simulink model "Controller"  (Simulink 10.0)
settings: Solver=FixedStepAuto  StartTime=0.0  StopTime=10.0  RelTol=1e-3
values from neighbouring files (symbols this model uses):
  Controlador = Simulink.Parameter    [Param_Controller.m]
  userParameters = Simulink.Parameter    [Param_Controller.m]
undefined symbols (not defined in the file or in its folder): Controlador_Curva, controllerGainsCurve, ControllerState_t, filter_r_den, filter_r_num, filter_r_Ts
libraries: simulink x8
settings Model: Creator=renan  LastModifiedBy=renan
settings DataIOCC: SaveFormat=Dataset  ReturnWorkspaceOutputs=on
settings OptimizationCC: DefaultParameterBehavior=Inlined  UseFloatMulNetSlope=on  DefaultUnderspecifiedDataType=single  PassReuseOutputArgsAs=Individual arguments  LifeSpan=auto  OptimizationLevel=level1  OptimizationPriority=Speed  MultiThreadedLoops=on  EfficientTunableParamExpr=on
settings DebuggingCC: UnderspecifiedInitializationDetection=Simplified  MergeDetectMultiDrivingBlocksExec=error  ParameterTunabilityLossMsg=error  SFUnexpectedBacktrackingDiag=error  SFNoUnconditionalDefaultTransitionDiag=error  SFExecutionAtInitializationDiag=warning  ArithmeticOperatorsInVariantConditions=error
settings HardwareCC: ProdBitPerPointer=64  ProdBitPerSizeT=64  ProdBitPerPtrDiffT=64  ProdLargestAtomicFloat=Float  ProdIntDivRoundTo=Zero  ProdEndianess=LittleEndian  ProdWordSize=64  ProdLongLongMode=on  ProdHWDeviceType=Intel->x86-64 (Windows64)
settings ModelReferenceCC: PropagateSignalLabelsOutOfModel=on
settings SFSimCC: SimUseLocalCustomCode=on  MATLABDynamicMemAlloc=off  CustomCodeUndefinedFunction=FilterOut
settings RTWCC: Description=Embedded Coder  SystemTargetFile=ert.tlc  TemplateMakefile=ert_default_tmf  GenerateReport=on  RTWUseLocalCustomCode=on  Toolchain=MinGW64 | gmake (64-bit Windows)  IncludeHyperlinkInReport=on  LaunchReport=on  TargetLang=C++  GenerateTraceInfo=on  GenerateTraceReport=on  GenerateTraceReportSl=on  GenerateTraceReportSf=on  GenerateTraceReportEml=on
settings CodeAppCC: ForceParamTrailComments=on  IgnoreCustomStorageClasses=off  OperatorAnnotations=on  SimulinkDataObjDesc=on  SFDataObjDesc=on  InsertBlockDesc=on  StateflowObjectComments=off
settings ERTTargetCC: TargetLangStandard=C++03 (ISO)  GenerateSampleERTMain=on  SuppressErrorStatus=on  MultiInstanceERTCode=on  CodeInterfacePackaging=C++ class  SupportNonFinite=off  SupportComplex=off  RootIOFormat=Structure reference  ERTCustomFileTemplate=example_file_process.tlc
settings CPPComponent: GenerateDestructor=on  GenerateExternalIOAccessMethods=None  ParameterMemberVisibility=public  InternalMemberVisibility=private  GenerateParameterAccessMethods=None  GenerateInternalMemberAccessMethods=None  UseOperatorNewForModelRefRegistration=off
settings ConfigComp: CovMetricSettings=dwe  CovHtmlReporting=off  CovSaveCumulativeToWorkspaceVar=off  CovSaveSingleToWorkspaceVar=off

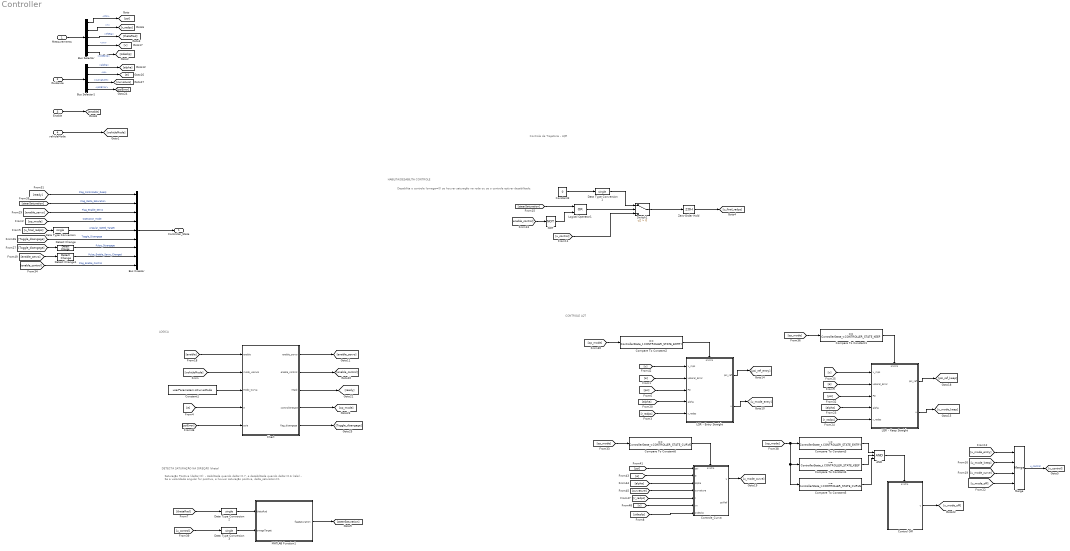
== system Controller ==
  note: DETECTA SATURAÇÃO NA DIREÇÃO (theta)
  note: LOGICA
  note: Desabilita o controle (omega=0) se houver saturação na roda ou se o controle estiver desabilitado.
  note: Controle de Trajetória - LQR
  note: Saturação Positiva (delta>0):
      | - Habilitada quando delta>0.7, e desabilitada quando delta<0.6 (relé)
      | - Se a velocidade angular for positiva, e houver saturação positiva, delta_saturation=1
  note: CONTROLE LQT
  note: HABILITA/DESABILITA CONTROLE
  Measurements : Inport  OutDataTypeStr=Bus: controllerMeasurementBus_t
  Guidance : Inport  Port=2  OutDataTypeStr=Bus: controllerInputGuidanceBus_t
  Enable : Inport  Port=3  OutDataTypeStr=boolean
  vehicleMode : Inport  Port=4  OutDataTypeStr=Enum: VehicleMode_t
  AND : Logic  Inputs=3  IconShape=distinctive  AllPortsSameDT=off  OutDataTypeStr=boolean
  Bus Creator : BusCreator  Inputs=9  OutDataTypeStr=Bus: Controler_Bus  NonVirtualBus=on
  Bus Selector : BusSelector  OutputSignals=Psi,r,theta,vx,sideslip
  Bus Selector1 : BusSelector  OutputSignals=alpha,e,curvature,psiError
  Chart : Stateflow chart  BlockKeywords=__PRM__SERIALIZED__DATA__:Stateflow Chart,Stateflow Diagram  TreatAsAtomicUnit=on
  Compare To Constant1 : simulink/Logic and Bit Operations/Compare To Constant  relop===  const=ControllerState_t.CONTROLLER_STATE_KEEP  OutDataTypeStr=boolean
  Compare To Constant2 : simulink/Logic and Bit Operations/Compare To Constant  relop===  const=ControllerState_t.CONTROLLER_STATE_ENTRY  OutDataTypeStr=boolean
  Compare To Constant3 : simulink/Logic and Bit Operations/Compare To Constant  relop=~=  const=ControllerState_t.CONTROLLER_STATE_ENTRY  OutDataTypeStr=boolean
  Compare To Constant4 : simulink/Logic and Bit Operations/Compare To Constant  relop=~=  const=ControllerState_t.CONTROLLER_STATE_KEEP  OutDataTypeStr=boolean
  Compare To Constant5 : simulink/Logic and Bit Operations/Compare To Constant  relop=~=  const=ControllerState_t.CONTROLLER_STATE_CURVE  OutDataTypeStr=boolean
  Compare To Constant6 : simulink/Logic and Bit Operations/Compare To Constant  relop===  const=ControllerState_t.CONTROLLER_STATE_CURVE  OutDataTypeStr=boolean
  Constant1 : Constant  Value=userParameters.isCurveMode
  Constant3 : Constant  Value=0
  Control Off : Subsystem  TreatAsAtomicUnit=on
  Controle_Curva : Subsystem  TreatAsAtomicUnit=on
  Data Type Conversion{,1..3} (4 alike) : DataTypeConversion  OutDataTypeStr=single
  Detect Change : simulink/Logic and Bit Operations/Detect Change  vinit=0  OutDataTypeStr=boolean
  Detect Change1 : simulink/Logic and Bit Operations/Detect Change  vinit=0  OutDataTypeStr=boolean
  LQR - Entry Straight : Subsystem  TreatAsAtomicUnit=on
  LQR - Keep Straight : Subsystem  TreatAsAtomicUnit=on
  Logical Operator1 : Logic  Operator=OR  IconShape=distinctive  AllPortsSameDT=off  OutDataTypeStr=boolean
  MATLAB Function1 : MATLAB Function  TreatAsAtomicUnit=on
  Merge : Merge  Inputs=4  InitialOutput=0
  NOT : Logic  Operator=NOT  IconShape=distinctive  AllPortsSameDT=off  OutDataTypeStr=boolean
  Switch1 : Switch  Criteria=u2 > Threshold
  Zero-Order Hold : ZeroOrderHold  SampleTime=0.05
  Controller_State : Outport  OutDataTypeStr=Bus: Controler_Bus
  wires:
  [r_radps] -> LQR - Entry Straight/5(r_radps)
  Compare To Constant5/1 -> AND/3
  [psiError] -> Chart/5(psie)
  [u_mode_keep] -> Merge/2
  LQR - Keep Straight/2(u) -> [u_mode_keep]
  Compare To Constant4/1 -> AND/2
  [Toggle_disengage] -> Detect Change/1
  [v] -> Controle_Curva/6(vx)
  Detect Change1/1 -> Bus Creator/8  "Pulse_Enable_Servo_Changed"
  Detect Change/1 -> Bus Creator/7  "Pulse_Disengage"
  LQR - Entry Straight/2(u) -> [u_mode_entry]
  [Toggle_disengage] -> Bus Creator/6  "Toggle_Disengage"
  [enable_servo] -> Detect Change1/1
  [enable_servo] -> Bus Creator/3  "Flag_Enable_Servo"
  Merge/1 -> [u_control]  "u_control"
  Chart/3(ready) -> [ready]
  [r_radps] -> Controle_Curva/5(r)
  [op_mode] -> Bus Creator/4  "Operation_Mode"
  [u_final_radps] -> Data Type Conversion/1
  [alpha] -> Controle_Curva/3(alpha)
  [psi] -> Controle_Curva/1(psi)
  Data Type Conversion/1 -> Bus Creator/5  "Angular_Speed_Target"
  [e] -> Controle_Curva/2(e)
  [op_mode] -> Compare To Constant6/1
  [steerSaturation] -> Bus Creator/2  "Flag_Delta_Saturation"
  Compare To Constant3/1 -> AND/1
  Bus Creator/1 -> Controller_State/1
  Compare To Constant2/1 -> LQR - Entry Straight/Enable
  Constant1/1 -> Chart/3(Modo_Curva)
  [u_control] -> Switch1/3
  [u_mode_entry] -> Merge/1
  [u_mode_off] -> Merge/4
  [e] -> Chart/4(e)
  [e] -> LQR - Entry Straight/2(Lateral_Error)
  Control Off/1(u) -> [u_mode_off]
  [ready] -> Bus Creator/1  "Flag_Controlador_Ready"
  Chart/5(flag_disengage) -> [Toggle_disengage]
  [psi] -> LQR - Entry Straight/3(Psi)
  [u_mode_curve] -> Merge/3
  Compare To Constant6/1 -> Controle_Curva/Enable
  LQR - Entry Straight/1(psi_ref) -> [psi_ref_entry]
  Switch1/1 -> Zero-Order Hold/1
  [v] -> LQR - Entry Straight/1(v_mps)
  Compare To Constant1/1 -> LQR - Keep Straight/Enable
  [psi] -> LQR - Keep Straight/3(Psi)
  AND/1 -> Control Off/Enable
  [op_mode] -> Compare To Constant5/1, Compare To Constant4/1, Compare To Constant3/1
  [r_radps] -> LQR - Keep Straight/5(r_radps)
  [v] -> LQR - Keep Straight/1(v_mps)
  [e] -> LQR - Keep Straight/2(Lateral_Error)
  [alpha] -> LQR - Entry Straight/4(alpha)
  [op_mode] -> Compare To Constant1/1
  [steerSaturation] -> Logical Operator1/1
  [op_mode] -> Compare To Constant2/1
  Controle_Curva/1(u) -> [u_mode_curve]
  Logical Operator1/1 -> Switch1/2
  Chart/1(enable_servo) -> [enable_servo]
  [curvature] -> Controle_Curva/4(curvature)
  [alpha] -> LQR - Keep Straight/4(alpha)
  Chart/4(controllerState) -> [op_mode]
  Chart/2(enable_control) -> [enable_control]
  NOT/1 -> Logical Operator1/2
  Constant3/1 -> Data Type Conversion1/1
  [enable] -> Chart/1(enable)
  LQR - Keep Straight/1(psi_ref) -> [psi_ref_keep]
  [enable_control] -> NOT/1
  Bus Selector/1 -> [psi]  "<Psi>"
  Bus Selector/2 -> [r_radps]  "<r>"
  Bus Selector/3 -> [thetaRad]  "<theta>"
  Bus Selector/4 -> [v]  "<vx>"
  Guidance/1 -> Bus Selector1/1
  Bus Selector1/1 -> [alpha]  "<alpha>"
  Bus Selector1/2 -> [e]  "<e>"
  Bus Selector1/3 -> [curvature]  "<curvature>"
  [enable_control] -> Bus Creator/9  "Flag_Enable_Control"
  Data Type Conversion1/1 -> Switch1/1
  Zero-Order Hold/1 -> [u_final_radps]
  MATLAB Function1/1(flagSaturation) -> [steerSaturation]
  [thetaRad] -> Data Type Conversion2/1
  [u_control] -> Data Type Conversion3/1
  Data Type Conversion2/1 -> MATLAB Function1/1(thetaRad)
  Data Type Conversion3/1 -> MATLAB Function1/2(omegaTarget)
  Bus Selector1/4 -> [psiError]  "<psiError>"
  Enable/1 -> [enable]
  vehicleMode/1 -> [vehicleMode]
  [vehicleMode] -> Chart/2(modo_veiculo)
  Measurements/1 -> Bus Selector/1
  Bus Selector/5 -> [sideslip]  "<sideslip>"
  [sideslip] -> Controle_Curva/7(sideslip)

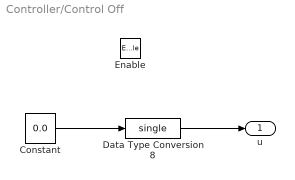
== system Controller/Control Off ==
  Enable : EnablePort
  Constant : Constant  Value=0.0  OutDataTypeStr=single  SampleTime=-1
  Data Type Conversion8 : DataTypeConversion  OutDataTypeStr=single
  u : Outport
  wires:
  Constant/1 -> Data Type Conversion8/1
  Data Type Conversion8/1 -> u/1

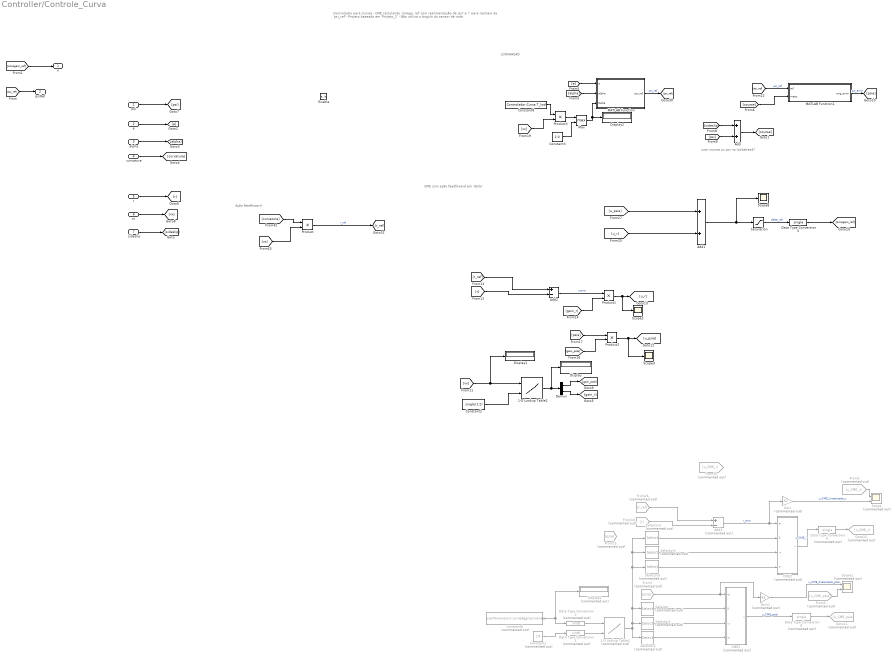
== system Controller/Controle_Curva ==
  note: usar course ou psi no lookahead?
  note: Controlador para Curvas
      |
      | - CME calculando 'omega_ref' com realimentação de 'psi' e 'r' para rastreio de 'psi_ref'
      | - Projeto baseado em 'Projeto_2'
      | - Não utiliza o ângulo do sensor de roda
  note: LOOKAHEAD
  note: CME com ação feedfoward em 'delta'
  note: Ação feedfoward
  psi : Inport  OutDataTypeStr=single  PortDimensions=1
  e : Inport  Port=2  OutDataTypeStr=single  PortDimensions=1
  alpha : Inport  Port=3  OutDataTypeStr=single  PortDimensions=1
  curvature : Inport  Port=4  OutDataTypeStr=single  PortDimensions=1
  r : Inport  Port=5  OutDataTypeStr=single  PortDimensions=1
  vx : Inport  Port=6  OutDataTypeStr=single  PortDimensions=1
  sideslip : Inport  Port=7
  Enable : EnablePort
  1-D Lookup Table1 : Lookup_n-D  Commented=on  BreakpointsForDimension1=uint8(1:7)  BreakpointsForDimension2=uint8(1:8)  IndexSearchMethod=Linear search  BeginIndexSearchUsingPreviousIndexResult=on  Table=controllerGainsCurve  ExtrapMethod=Clip  UseLastTableValue=on  InternalRulePriority=Speed  OutDataTypeStr=single  RndMeth=Simplest  InputSameDT=on
  1-D Lookup Table2 : Lookup_n-D  BreakpointsForDimension1=Controlador.Curva.v_index  BreakpointsForDimension2=uint8(1:2)  IndexSearchMethod=Linear search  BeginIndexSearchUsingPreviousIndexResult=on  Table=Controlador.Curva.Gains  ExtrapMethod=Clip  UseLastTableValue=on  InternalRulePriority=Speed  OutDataTypeStr=single  RndMeth=Simplest  InputSameDT=on
  Add : Sum
  Add1 : Sum
  Add2 : Sum  Inputs=+-
  Add3 : Sum  Commented=on  Inputs=+-
  CME1 : MATLAB Function  Commented=on  TreatAsAtomicUnit=on
  CME2 : MATLAB Function  Commented=on  TreatAsAtomicUnit=on
  Constant1 : Constant  Commented=on  Value=1:8
  Constant2 : Constant  Value=single(1:2)
  Constant3 : Constant  Value=2.0
  Constant6 : Constant  Commented=on  Value=userParameters.curveAggressiveness
  Constant8 : Constant  Value=Controlador.Curva.T_look  SampleTime=-1
  Data Type Conversion1 : DataTypeConversion  Commented=on  OutDataTypeStr=uint8
  Data Type Conversion2 : DataTypeConversion  Commented=on  OutDataTypeStr=uint8
  Data Type Conversion3 : DataTypeConversion  OutDataTypeStr=single
  Data Type Conversion8 : DataTypeConversion  Commented=on  OutDataTypeStr=single
  Data Type Conversion9 : DataTypeConversion  Commented=on  OutDataTypeStr=single
  Demux : Demux  Outputs=2
  Display : Display
  Display1 : Display
  Display2 : Display
  Display4 : Display  Commented=on
  From15 : From  Commented=on  GotoTag=psie
  From16 : From  Commented=on  GotoTag=r
  From2 : From  Commented=on  GotoTag=u_CME_r
  From20 : From  Commented=on  GotoTag=u_CME_r
  From26 : From  Commented=on  GotoTag=r_ref
  From3 : From  Commented=on  GotoTag=u_CME_psie
  From7 : From  Commented=on  GotoTag=psie
  Gain : Gain  Commented=on  Gain=52
  Gain1 : Gain  Commented=on  Gain=43
  Goto11 : Goto  Commented=on  GotoTag=u_CME_psie
  Goto15 : Goto  Commented=on  GotoTag=u_CME_r
  MATLAB Function : MATLAB Function  TreatAsAtomicUnit=on
  MATLAB Function1 : MATLAB Function  TreatAsAtomicUnit=on
  Max : MinMax  Function=max  Inputs=2
  Product{,1..3} (4 alike) : Product
  Saturation : Saturate  UpperLimit=Controlador.Curva.omegam_sat  LowerLimit=-Controlador.Curva.omegam_sat
  Scope : Scope  Commented=on  NumInputPorts=2
  Scope1 : Scope  Commented=on  NumInputPorts=2
  Scope2 : Scope
  Scope3 : Scope
  Scope8 : Scope
  Selector : Selector  Commented=on  InputPortWidth=8  IndexOptions=Index vector (dialog)  Indices=[2]  OutputSizes=1
  Selector1 : Selector  Commented=on  InputPortWidth=8  IndexOptions=Index vector (dialog)  Indices=[3 4]  OutputSizes=1
  Selector2 : Selector  Commented=on  InputPortWidth=8  IndexOptions=Index vector (dialog)  Indices=[1]  OutputSizes=1
  Selector3 : Selector  Commented=on  InputPortWidth=8  IndexOptions=Index vector (dialog)  Indices=[6]  OutputSizes=1
  Selector4 : Selector  Commented=on  InputPortWidth=8  IndexOptions=Index vector (dialog)  Indices=[7 8]  OutputSizes=1
  Selector5 : Selector  Commented=on  InputPortWidth=8  IndexOptions=Index vector (dialog)  Indices=[5]  OutputSizes=1
  u : Outport
  psiRef : Outport  Port=2
  wires:
  [psi_ref] -> MATLAB Function1/1(ref)  "psi_ref"
  MATLAB Function/1(psi_ref) -> [psi_ref]  "psi_ref"
  MATLAB Function1/1(ang_error) -> [psie]  "psi_error"
  [e] -> MATLAB Function/1(e)
  [alpha] -> MATLAB Function/2(alpha)
  Add1/1 -> Scope8/1, Saturation/1
  CME2/1(u) -> Data Type Conversion9/1  "u_CME_r"
  CME1/1(u) -> Data Type Conversion8/1  "u_CME_psie"
  From26/1 -> Add3/1
  From16/1 -> Add3/2
  Saturation/1 -> Data Type Conversion3/1  "delta_ref"
  Product/1 -> [r_ref]  "r_ref"
  [curvature] -> Product/1
  [vx] -> Product/2
  psi/1 -> [psi]
  e/1 -> [e]
  alpha/1 -> [alpha]
  curvature/1 -> [curvature]
  r/1 -> [r]
  Add3/1 -> Gain/1, CME2/1(et)  "r_erro"
  [omegam_ref] -> u/1
  vx/1 -> [vx]
  From7/1 -> CME1/1(et), Gain1/1
  Selector/1 -> CME1/2(B)
  Selector1/1 -> CME1/3(ur)
  Selector2/1 -> CME1/4(er)
  Selector3/1 -> CME2/2(B)
  Selector4/1 -> CME2/3(ur)
  Selector5/1 -> CME2/4(er)
  Data Type Conversion8/1 -> Goto11/1
  Data Type Conversion9/1 -> Goto15/1
  Gain/1 -> Scope/2  "u_CME_Linearizado_r"
  Gain1/1 -> Scope1/1  "u_CME_linearizado_psie"
  Constant6/1 -> Display4/1, Data Type Conversion2/1
  Constant1/1 -> Data Type Conversion1/1
  1-D Lookup Table1/1 -> Selector3/1, Selector4/1, Selector5/1, Selector/1, Selector1/1, Selector2/1
  Data Type Conversion2/1 -> 1-D Lookup Table1/1
  Data Type Conversion1/1 -> 1-D Lookup Table1/2
  [psi_ref] -> psiRef/1
  From2/1 -> Scope/1
  From3/1 -> Scope1/2
  sideslip/1 -> [sideslip]
  [sideslip] -> Add/1
  [psi] -> Add/2
  Add/1 -> [course]
  [vx] -> Display1/1, 1-D Lookup Table2/1
  Constant2/1 -> 1-D Lookup Table2/2
  1-D Lookup Table2/1 -> Display/1, Demux/1
  Demux/1 -> [gain_psie]
  Demux/2 -> [gain_r]
  [r_ref] -> Add2/1
  Add2/1 -> Product1/1  "r_erro"
  [r] -> Add2/2
  [psie] -> Product2/1
  Product2/1 -> Scope3/1, [u_psie]
  Product1/1 -> Scope2/1, [u_r]
  Constant8/1 -> Product3/1
  [vx] -> Product3/2
  Product3/1 -> Max/1
  Max/1 -> Display2/1, MATLAB Function/3(Delta)
  Constant3/1 -> Max/2
  [u_psie] -> Add1/1
  [u_r] -> Add1/2
  [gain_psie] -> Product2/2
  [gain_r] -> Product1/2
  [course] -> MATLAB Function1/2(meas)
  Data Type Conversion3/1 -> [omegam_ref]

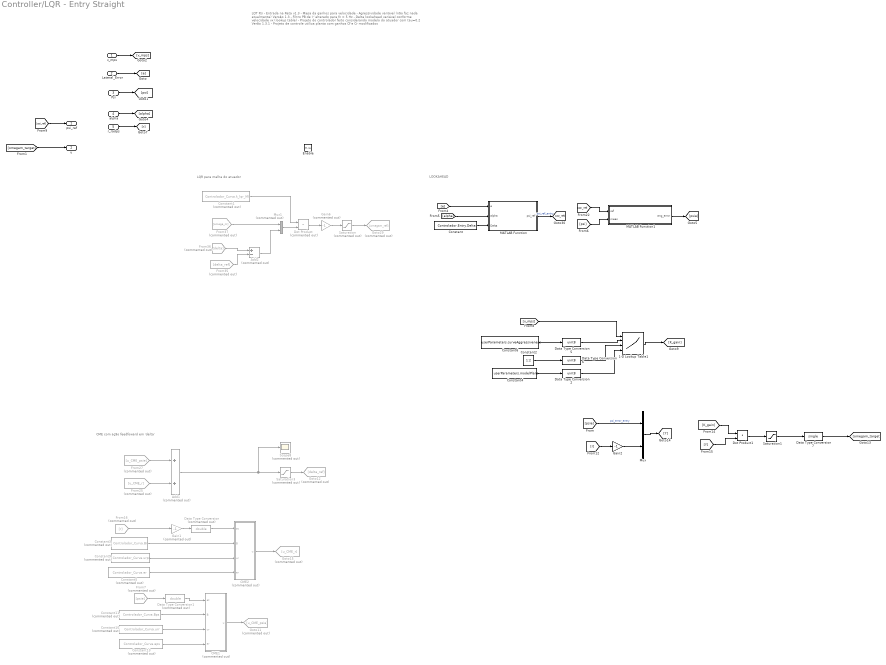
== system Controller/LQR - Entry Straight ==
  note: LQT Psi - Entrada na Reta v1.3
      | - Mapa da ganhos para velocidade
      | - Agressividade variável (não faz nada atualmente)
      |
      | Versão 1.3
      | - Filtro PB de 'r' alterado para fc = 5 Hz
      | - Delta lookahead variável conforme velocidade vx (lookup table)
      | - Projeto do controlador feito considerando modelo do atuador com tau=0.2
      |
      | Verão 1.3.1
      | - Projeto de controle utiliza planta com ganhos Cf e Cr modificados
  note: LQR para malha do atuador
  note: LOOKAHEAD
  note: CME com ação feedfoward em 'delta'
  v_mps : Inport  OutDataTypeStr=single  PortDimensions=1
  Lateral_Error : Inport  Port=2  PortDimensions=1
  Psi : Inport  Port=3  PortDimensions=1
  alpha : Inport  Port=4  PortDimensions=1
  r_radps : Inport  Port=5  PortDimensions=1
  Enable : EnablePort
  1-D Lookup Table1 : Lookup_n-D  NumberOfTableDimensions=4  BreakpointsForDimension1=Controlador.Entry.v_index  BreakpointsForDimension2=uint8(1:7)  BreakpointsForDimension3=uint8(1:2)  BreakpointsForDimension4=uint8(1:2)  IndexSearchMethod=Linear search  BeginIndexSearchUsingPreviousIndexResult=on  Table=Controlador.Entry.Gains  TableDataTypeStr=Inherit: Inherit from 'Table data'  ExtrapMethod=Clip  UseLastTableValue=on  InternalRulePriority=Speed  OutDataTypeStr=Inherit: Inherit from 'Table data'  RndMeth=Simplest
  Add1 : Sum  Commented=on
  Add2 : Sum  Commented=on  Inputs=+-
  CME1 : MATLAB Function  Commented=on  TreatAsAtomicUnit=on
  CME2 : MATLAB Function  Commented=on  TreatAsAtomicUnit=on
  Constant : Constant  Value=Controlador.Entry.Delta
  Constant1 : Constant  Commented=on  Value=Controlador_Curva.k_lqr_MI  VectorParams1D=off  SampleTime=-1
  Constant10 : Constant  Commented=on  Value=Controlador_Curva.urr  VectorParams1D=off  SampleTime=-1
  Constant11 : Constant  Commented=on  Value=Controlador_Curva.Bps  SampleTime=-1
  Constant13 : Constant  Commented=on  Value=Controlador_Curva.eps  SampleTime=-1
  Constant2 : Constant  Value=1:2
  Constant3 : Constant  Commented=on  Value=Controlador_Curva.Br  SampleTime=-1
  Constant4 : Constant  Value=userParameters.modelPlant
  Constant5 : Constant  Commented=on  Value=Controlador_Curva.er  SampleTime=-1
  Constant6 : Constant  Value=userParameters.curveAggressiveness
  Constant9 : Constant  Commented=on  Value=Controlador_Curva.urps  VectorParams1D=off  SampleTime=-1
  Data Type Conversion : DataTypeConversion  Commented=on  OutDataTypeStr=double
  Data Type Conversion1 : DataTypeConversion  Commented=on  OutDataTypeStr=double
  Data Type Conversion2 : DataTypeConversion  OutDataTypeStr=uint8
  Data Type Conversion5 : DataTypeConversion  OutDataTypeStr=uint8
  Data Type Conversion6 : DataTypeConversion  OutDataTypeStr=uint8
  Data Type Conversion7 : DataTypeConversion  OutDataTypeStr=single
  Dot Product : DotProduct  Commented=on  InputSameDT=on  OutDataTypeStr=Inherit: Inherit via internal rule
  Dot Product1 : DotProduct  InputSameDT=on  OutDataTypeStr=Inherit: Inherit via internal rule
  From16 : From  Commented=on  GotoTag=r
  From25 : From  Commented=on  GotoTag=u_CME_r
  From27 : From  Commented=on  GotoTag=u_CME_psie
  From35 : From  Commented=on  GotoTag=delta_ref
  From36 : From  Commented=on  GotoTag=delta
  From37 : From  Commented=on  GotoTag=omega_m
  From7 : From  Commented=on  GotoTag=psie
  Gain1 : Gain  Commented=on  Gain=-1
  Gain2 : Gain  Gain=-1
  Gain6 : Gain  Commented=on  Gain=-1
  Goto11 : Goto  Commented=on  GotoTag=u_CME_psie
  Goto12 : Goto  Commented=on  GotoTag=delta_ref
  Goto15 : Goto  Commented=on  GotoTag=u_CME_r
  Goto29 : Goto  Commented=on  GotoTag=omegam_ref
  MATLAB Function : MATLAB Function  TreatAsAtomicUnit=on
  MATLAB Function1 : MATLAB Function  TreatAsAtomicUnit=on
  Mux : Mux  Inputs=2
  Mux1 : Mux  Commented=on  Inputs=2
  Saturation : Saturate  Commented=on  UpperLimit=4  LowerLimit=-4
  Saturation1 : Saturate  UpperLimit=Controlador.Entry.omegam_sat  LowerLimit=-Controlador.Entry.omegam_sat
  Saturation3 : Saturate  Commented=on  UpperLimit=0.8  LowerLimit=-0.8
  Scope8 : Scope  Commented=on
  psi_ref : Outport
  u : Outport  Port=2
  wires:
  v_mps/1 -> [v_mps]
  Lateral_Error/1 -> [e]
  Psi/1 -> [psi]
  alpha/1 -> [alpha]
  r_radps/1 -> [r]
  [psi_ref] -> psi_ref/1
  [e] -> MATLAB Function/1(e)
  From35/1 -> Add2/2
  Add2/1 -> Mux1/2
  Constant10/1 -> CME1/3(ur)
  Data Type Conversion/1 -> CME2/1(et)
  Saturation3/1 -> Goto12/1
  Mux1/1 -> Dot Product/2
  Constant3/1 -> CME2/2(B)
  Gain6/1 -> Saturation/1
  Dot Product/1 -> Gain6/1
  From37/1 -> Mux1/1
  From36/1 -> Add2/1
  Constant9/1 -> CME2/3(ur)
  Saturation/1 -> Goto29/1
  From27/1 -> Add1/1
  Constant11/1 -> CME1/2(B)
  Constant1/1 -> Dot Product/1
  From16/1 -> Gain1/1
  Add1/1 -> Scope8/1, Saturation3/1
  Data Type Conversion1/1 -> CME1/1(et)
  From7/1 -> Data Type Conversion1/1
  From25/1 -> Add1/2
  [psi] -> MATLAB Function1/2(meas)
  Constant5/1 -> CME2/4(er)
  Constant/1 -> MATLAB Function/3(Delta)
  MATLAB Function1/1(ang_error) -> [psie]
  MATLAB Function/1(psi_ref) -> [psi_ref]  "psi_ref_entry"
  Constant13/1 -> CME1/4(er)
  [alpha] -> MATLAB Function/2(alpha)
  [psi_ref] -> MATLAB Function1/1(ref)
  CME2/1(u) -> Goto15/1
  CME1/1(u) -> Goto11/1
  Gain1/1 -> Data Type Conversion/1
  [omegam_target] -> u/1
  Constant4/1 -> Data Type Conversion2/1
  Dot Product1/1 -> Saturation1/1
  Mux/1 -> [Y]
  [psie] -> Mux/1  "psi_error_entry"
  Gain2/1 -> Mux/2
  [K_gain] -> Dot Product1/1
  Data Type Conversion7/1 -> [omegam_target]
  [r] -> Gain2/1
  [Y] -> Dot Product1/2
  Data Type Conversion2/1 -> 1-D Lookup Table1/4
  [v_mps] -> 1-D Lookup Table1/1
  Data Type Conversion6/1 -> 1-D Lookup Table1/3
  Saturation1/1 -> Data Type Conversion7/1
  Constant2/1 -> Data Type Conversion6/1
  Data Type Conversion5/1 -> 1-D Lookup Table1/2
  Constant6/1 -> Data Type Conversion5/1
  1-D Lookup Table1/1 -> [K_gain]

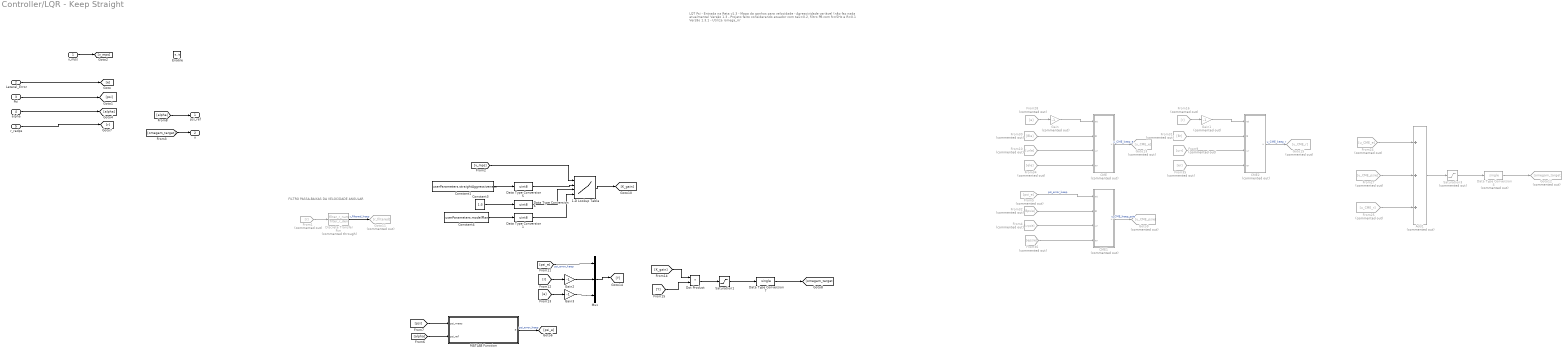
== system Controller/LQR - Keep Straight ==
  note: FILTRO PASSA-BAIXAS DA VELOCIDADE ANGULAR
  note: LQT Psi - Entrada na Reta v1.3
      | - Mapa da ganhos para velocidade
      | - Agressividade variável (não faz nada atualmente)
      |
      | Versão 1.3
      | - Projeto feito considerando atuador com tau=0.2, filtro PB com fc=5Hz e R=0.1
      |
      | Versão 1.3.1
      | - Utiliza 'omega_m'
  v_mps : Inport  OutDataTypeStr=single  PortDimensions=1
  Lateral_Error : Inport  Port=2  PortDimensions=1
  Psi : Inport  Port=3  PortDimensions=1
  alpha : Inport  Port=4  PortDimensions=1
  r_radps : Inport  Port=5  PortDimensions=1
  Enable : EnablePort
  1-D Lookup Table : Lookup_n-D  NumberOfTableDimensions=4  BreakpointsForDimension1=Controlador.Keep.v_index  BreakpointsForDimension2=uint8(1:7)  BreakpointsForDimension3=uint8(1:3)  BreakpointsForDimension4=uint8(1:4)  IndexSearchMethod=Linear search  BeginIndexSearchUsingPreviousIndexResult=on  Table=Controlador.Keep.Gains  TableDataTypeStr=Inherit: Inherit from 'Table data'  ExtrapMethod=Clip  UseLastTableValue=on  InternalRulePriority=Speed  OutDataTypeStr=Inherit: Inherit from 'Table data'  RndMeth=Simplest
  Add1 : Sum  Commented=on  Inputs=+++
  CME : MATLAB Function  Commented=on  TreatAsAtomicUnit=on
  CME1 : MATLAB Function  Commented=on  TreatAsAtomicUnit=on
  CME2 : MATLAB Function  Commented=on  TreatAsAtomicUnit=on
  Constant1 : Constant  Value=userParameters.straightAggressiveness
  Constant3 : Constant  Value=1:3
  Constant4 : Constant  Value=userParameters.modelPlant
  Data Type Conversion1 : DataTypeConversion  OutDataTypeStr=uint8
  Data Type Conversion4 : DataTypeConversion  Commented=on  OutDataTypeStr=single
  Data Type Conversion5 : DataTypeConversion  OutDataTypeStr=uint8
  Data Type Conversion6 : DataTypeConversion  OutDataTypeStr=uint8
  Data Type Conversion7 : DataTypeConversion  OutDataTypeStr=single
  Discrete Transfer Fcn : DiscreteTransferFcn  Commented=through  Numerator=filter_r_num  Denominator=filter_r_den  SampleTime=filter_r_Ts
  Dot Product : DotProduct  InputSameDT=on  OutDataTypeStr=Inherit: Inherit via internal rule
  From1 : From  Commented=on  GotoTag=r
  From10 : From  Commented=on  GotoTag=urle
  From16 : From  Commented=on  GotoTag=r
  From24 : From  Commented=on  GotoTag=u_CME_e
  From25 : From  Commented=on  GotoTag=u_CME_r
  From27 : From  Commented=on  GotoTag=u_CME_psie
  From28 : From  Commented=on  GotoTag=e
  From30 : From  Commented=on  GotoTag=Ble
  From31 : From  Commented=on  GotoTag=Br
  From32 : From  Commented=on  GotoTag=Bpsie
  From34 : From  Commented=on  GotoTag=ele
  From35 : From  Commented=on  GotoTag=er
  From36 : From  Commented=on  GotoTag=epsie
  From4 : From  Commented=on  GotoTag=urpsie
  From5 : From  Commented=on  GotoTag=psi_e
  From9 : From  Commented=on  GotoTag=urr
  Gain : Gain  Commented=on  Gain=-1
  Gain1 : Gain  Commented=on  Gain=-1
  Gain2 : Gain  Gain=-1
  Gain3 : Gain  Gain=-1
  Goto11 : Goto  Commented=on  GotoTag=r_filtered
  Goto12 : Goto  Commented=on  GotoTag=omegam_target
  Goto13 : Goto  Commented=on  GotoTag=u_CME_e
  Goto15 : Goto  Commented=on  GotoTag=u_CME_r
  Goto9 : Goto  Commented=on  GotoTag=u_CME_psie
  MATLAB Function : MATLAB Function  TreatAsAtomicUnit=on
  Mux : Mux  Inputs=3
  Saturation1 : Saturate  UpperLimit=Controlador.Keep.omegam_sat  LowerLimit=-Controlador.Keep.omegam_sat
  Saturation3 : Saturate  Commented=on  UpperLimit=Controlador.Keep.omegam_sat  LowerLimit=-Controlador.Keep.omegam_sat
  psi_ref : Outport
  u : Outport  Port=2
  wires:
  v_mps/1 -> [v_mps]
  [alpha] -> MATLAB Function/2(psi_ref)
  [psi] -> MATLAB Function/1(psi_meas)
  MATLAB Function/1(e) -> [psi_e]  "psi_error_keep"
  From1/1 -> Discrete Transfer Fcn/1
  Discrete Transfer Fcn/1 -> Goto11/1  "r_filtered_keep"
  [alpha] -> psi_ref/1
  [omegam_target] -> u/1
  From5/1 -> CME1/1(et)  "psi_error_keep"
  From36/1 -> CME1/4(er)
  From31/1 -> CME2/2(B)
  Gain1/1 -> CME2/1(et)
  CME1/1(u) -> Goto9/1  "u_CME_keep_psie"
  From9/1 -> CME2/3(ur)
  Constant1/1 -> Data Type Conversion5/1
  From4/1 -> CME1/3(ur)
  Saturation3/1 -> Data Type Conversion4/1
  Add1/1 -> Saturation3/1
  From27/1 -> Add1/2
  From24/1 -> Add1/1
  From28/1 -> Gain/1
  Constant3/1 -> Data Type Conversion6/1
  From32/1 -> CME1/2(B)
  CME2/1(u) -> Goto15/1  "u_CME_keep_r"
  Gain/1 -> CME/1(et)
  CME/1(u) -> Goto13/1  "u_CME_keep_e"
  From35/1 -> CME2/4(er)
  From25/1 -> Add1/3
  From30/1 -> CME/2(B)
  From10/1 -> CME/3(ur)
  From34/1 -> CME/4(er)
  From16/1 -> Gain1/1
  Lateral_Error/1 -> [e]
  Psi/1 -> [psi]
  alpha/1 -> [alpha]
  r_radps/1 -> [r]
  Data Type Conversion4/1 -> Goto12/1
  Data Type Conversion5/1 -> 1-D Lookup Table/2
  [v_mps] -> 1-D Lookup Table/1
  Data Type Conversion6/1 -> 1-D Lookup Table/3
  Data Type Conversion7/1 -> [omegam_target]
  Saturation1/1 -> Data Type Conversion7/1
  [psi_e] -> Mux/1  "psi_error_keep"
  [r] -> Gain2/1
  [e] -> Gain3/1
  1-D Lookup Table/1 -> [K_gain]
  Mux/1 -> [Y]
  Dot Product/1 -> Saturation1/1
  [Y] -> Dot Product/2
  [K_gain] -> Dot Product/1
  Gain2/1 -> Mux/2
  Gain3/1 -> Mux/3
  Constant4/1 -> Data Type Conversion1/1
  Data Type Conversion1/1 -> 1-D Lookup Table/4

== stateflow chart Chart ==
  settings: updateMethod=DISCRETE
  note: Inputs
      | Outputs
      | reset_integrator : Quando true, apaga o erro acumulado dos integradores.
      | enable_sm : Quando true, habilita a alimentação do motor de passo (sem necessariamente movimentá-lo). Quando false, libera a direção.
      | enable_control : Quando true, habilita o controlador. Quando false, a entrada dos integradores e a saída de atuação são nulas.
      | ready : Flag que indica que o controlador está atuando, ou está pronto para atuar. True nos estados ON e WAIT.
      |
      | States
      | CONTROL_OFF : E stado inicial. Controlador desligado, integrador resetado e motor desligado.
      | CONTROL_INIT: Motor é ligado. Para chegar neste estado, é necessário um enable e que o veículo esteja andando ou parado (sem ré)
      | CONTROL_WAIT: Controlador desligado e motor ligado. Só permanece neste estado se modo_veiculo=Parado e enable=true.
      | CONTROL_ON: Controlador e motor ligados. Só permanece neste estado se modo_veiculo=Andando e enable=true.
  state CONTROL_ON
    enable_control=true;
    ready = true;
    state MODE_ENTRY
      controllerState = CONTROLLER_STATE_ENTRY;
    state MODE_CURVE
      controllerState = CONTROLLER_STATE_CURVE;
    state MODE_KEEP
      controllerState = CONTROLLER_STATE_KEEP;
    MODE_ENTRY -> MODE_KEEP : [abs(e)<=0.15 && abs(psie)<=0.1]
  state CONTROL_OFF
    enable_servo = false;
    enable_control = false;
    ready = false;
    controllerState = CONTROLLER_STATE_IDLE;
  state CONTROL_WAIT
    enable_control = false;
    ready = true;
    controllerState = CONTROLLER_STATE_WAIT;
  state CONTROL_INIT
    enable_servo = true;
    controllerState = CONTROLLER_STATE_IDLE;
  CONTROL_WAIT -> MODE_ENTRY [order 4] : [~Modo_Curva]
  (default) -> CONTROL_OFF
  CONTROL_ON -> CONTROL_OFF [order 1] : [~enable]{flag_disengage=~flag_disengage}
  CONTROL_OFF -> CONTROL_OFF [order 1] : [modo_veiculo==VEHICLE_MODE_REVERSE || ~enable]
  CONTROL_WAIT -> MODE_CURVE [order 3] : [Modo_Curva]
  CONTROL_WAIT -> CONTROL_OFF [order 1] : [~enable || modo_veiculo==VEHICLE_MODE_REVERSE ]{flag_disengage=~flag_disengage}
  CONTROL_ON -> CONTROL_WAIT [order 2] : [modo_veiculo~=VEHICLE_MODE_FORWARD || hasChanged(Modo_Curva)]
  CONTROL_OFF -> CONTROL_INIT [order 2]
  CONTROL_INIT -> CONTROL_WAIT : [after(0.1, 'sec')]
  CONTROL_WAIT -> CONTROL_WAIT [order 2] : [modo_veiculo==VEHICLE_MODE_STOPPED ]
  data: enable input boolean size=1; enable_servo output boolean size=1; modo_veiculo input Enum: VehicleMode_t; enable_control output boolean size=1 =false; ready output boolean size=1 =false; controllerState output Enum: ControllerState_t size=1 =ControllerState_t.CONTROLLER_STATE_NONE; Modo_Curva input boolean size=1; e input double; flag_disengage output boolean =false; psie input double size=1

== matlab function Controle_Curva/MATLAB Function ==
  data: e input double; psi_ref output double; alpha input double; Delta input double
function psi_ref = Lookahead(e, alpha, Delta)

psi_ref = alpha + atan(-e/Delta);

== matlab function Controle_Curva/MATLAB Function1 ==
  data: ref input double; ang_error output double; meas input double
% ref-meas
function ang_error = Angular_Error(ref, meas)

    ref = mod(ref, 2*pi);
    meas = mod(meas, 2*pi);
    
    if(meas > ref)
        if(abs(2*pi-meas+ref) < abs(ref-meas))
            ang_error = 2*pi-meas+ref;
        else
            ang_error = ref - meas;
        end
    elseif (meas < ref)
        if(abs(meas - ref) < abs(2*pi-ref+meas))
            ang_error = ref - meas;
        else
            ang_error = -(meas + 2*pi - ref);
        end
    else
        ang_error = single(0);
    end
end

== matlab function Controle_Curva/CME1 ==
  data: u output single size=1; et input double size=1; B input double size=1; ur input double size=[2,1]; er input double size=1
% et: erro (ref-meas)
% B: Parâmetro 3
% ur: Parâmetro 2 (batentes do controle)
% er: Parâmetro
function u = CME(et, B, ur, er)


umin = ur(1); umax = ur(2);
% Cálculo do erro
%et = yref - y;
e = et / er;
if e < -1, e = single(-1);  elseif e > 1, e = single(1); end
% Cálculo de u
if abs(e) == 1, ut = e; else ss = e - sign(e); ut = sign(ss) * (abs(ss) ^ (2 ^ -B) - 1); end
% Cálculo da saída
a = (umax - umin) / 2; u = a * (ut - 1) + umax;

end

== matlab function LQR - Entry Straight/CME1 ==
  data: u output double size=1; et input double size=1; B input double size=1; ur input double size=[2,1]; er input double size=1
% et: erro (ref-meas)
% B: Parâmetro 3
% ur: Parâmetro 2 (batentes do controle)
% er: Parâmetro
function u = CME(et, B, ur, er)


umin = ur(1); umax = ur(2);
% Cálculo do erro
%et = yref - y;
e = et / er;
if e < -1, e = -1;  elseif e > 1, e = 1; end
% Cálculo de u
if abs(e) == 1, ut = e; else ss = e - sign(e); ut = sign(ss) * (abs(ss) ^ (2 ^ -B) - 1); end
% Cálculo da saída
a = (umax - umin) / 2; u = a * (ut - 1) + umax;

end

== matlab function Controle_Curva/CME2 ==
  data: u output double size=1; et input double size=1; B input double size=1; ur input double size=[2,1]; er input double size=1
% et: erro (ref-meas)
% B: Parâmetro 3
% ur: Parâmetro 2 (batentes do controle)
% er: Parâmetro
function u = CME(et, B, ur, er)


umin = ur(1); umax = ur(2);
% Cálculo do erro
%et = yref - y;

e = et / er;

if e < -1
    e = single(-1);
elseif e > 1
    e = single(1);
end

% Cálculo de u
if abs(e) == 1
    ut = e;
else
    ss = e - sign(e);
    ut = sign(ss) * (abs(ss) ^ (2 ^ -B) - 1);
end

% Cálculo da saída
a = (umax - umin) / 2; u = a * (ut - 1) + umax;

end

== matlab function LQR - Entry Straight/CME2 ==
  data: u output double size=1; et input double size=1; B input double size=1; ur input double size=[2,1]; er input double size=1
% et: erro (ref-meas)
% B: Parâmetro 3
% ur: Parâmetro 2 (batentes do controle)
% er: Parâmetro
function u = CME(et, B, ur, er)


umin = ur(1); umax = ur(2);
% Cálculo do erro
%et = yref - y;
e = et / er;
if e < -1, e = -1;  elseif e > 1, e = 1; end
% Cálculo de u
if abs(e) == 1, ut = e; else ss = e - sign(e); ut = sign(ss) * (abs(ss) ^ (2 ^ -B) - 1); end
% Cálculo da saída
a = (umax - umin) / 2; u = a * (ut - 1) + umax;

end

== matlab function MATLAB Function1 ==
  data: thetaRad input double; flagSaturation output double; omegaTarget input double; steerCalibration parameter double
function flagSaturation = fcn( thetaRad, omegaTarget, steerCalibration)

flagSaturation = false;

persistent rigthSaturation leftSaturation

if(isempty(rigthSaturation))
    rigthSaturation = false;
end

if(isempty(leftSaturation))
    leftSaturation = false;
end


if(steerCalibration.isCalibrated)
    
    % Relé da Saturação a direita
    % Menor o valor, mais a direita a roda está
    if(rigthSaturation)
        if(thetaRad > (steerCalibration.rightValue + steerCalibration.deadZone))
            rigthSaturation = false;
        end
    else
        if(thetaRad < steerCalibration.rightValue)
            rigthSaturation = true;
        end
    end
    
    % Relé da Saturação a esquerda
    % quanto maior o valor, mais a esquerda a roda está
    if(leftSaturation)

        if(thetaRad < (steerCalibration.leftValue - steerCalibration.deadZone))
            leftSaturation = false;
        end
    else
        if(thetaRad > steerCalibration.leftValue)
            leftSaturation = true;
        end
    end
    
    
    % Desliga a velocidade angular conforme saturação e sinal
    if((rigthSaturation && omegaTarget<0) || (leftSaturation && omegaTarget>0))
        flagSaturation = true;
    end

end


end

== matlab function LQR - Entry Straight/MATLAB Function ==
  data: e input double; psi_ref output double; alpha input double; Delta input double
function psi_ref = Lookahead(e, alpha, Delta)

psi_ref = alpha + atan(-e/Delta);

== matlab function LQR - Entry Straight/MATLAB Function1 ==
  data: ref input double; ang_error output double; meas input double
% ref-meas
function ang_error = Angular_Error(ref, meas)

    ref = mod(ref, 2*pi);
    meas = mod(meas, 2*pi);
    
    if(meas > ref)
        if(abs(2*pi-meas+ref) < abs(ref-meas))
            ang_error = 2*pi-meas+ref;
        else
            ang_error = ref - meas;
        end
    elseif (meas < ref)
        if(abs(meas - ref) < abs(2*pi-ref+meas))
            ang_error = ref - meas;
        else
            ang_error = -(meas + 2*pi - ref);
        end
    else
        ang_error = single(0);
    end
end

== matlab function LQR - Keep Straight/MATLAB Function ==
  data: psi_meas input double; e output double; psi_ref input double
% ref-meas
function e = Compute_Angular_Error(psi_meas, psi_ref)

psi_meas_ = mod(psi_meas, 2*pi);
psi_ref_ = mod(psi_ref, 2*pi);

if(psi_meas_ > psi_ref_)
    if(abs(2*pi-psi_meas_+psi_ref_) < abs(psi_ref_-psi_meas_))
        e = 2*pi-psi_meas_+psi_ref_;
    else
        e = psi_ref_ - psi_meas_;
    end
elseif (psi_meas_ < psi_ref_)
    if(abs(psi_meas_ - psi_ref_) < abs(2*pi-psi_ref_+psi_meas_))
        e = psi_ref_ - psi_meas_;
    else
        e = -(psi_meas_ + 2*pi - psi_ref_);
    end
else
    e = single(0);
end

end

== matlab function LQR - Keep Straight/CME ==
  data: u output double size=1; et input double size=1; B input double size=1; ur input double size=[2,1]; er input double size=1
% et: erro (ref-meas)
% B: Parâmetro 3
% ur: Parâmetro 2 (batentes do controle)
% er: Parâmetro
function u = CME(et, B, ur, er)


umin = ur(1); umax = ur(2);
% Cálculo do erro
%et = yref - y;
e = et / er;
if e < -1, e = -1;  elseif e > 1, e = 1; end
% Cálculo de u
if abs(e) == 1, ut = e; else ss = e - sign(e); ut = sign(ss) * (abs(ss) ^ (2 ^ -B) - 1); end
% Cálculo da saída
a = (umax - umin) / 2; u = a * (ut - 1) + umax;

end

== matlab function LQR - Keep Straight/CME1 ==
  data: u output double size=1; et input double size=1; B input double size=1; ur input double size=[2,1]; er input double size=1
% et: erro (ref-meas)
% B: Parâmetro 3
% ur: Parâmetro 2 (batentes do controle)
% er: Parâmetro
function u = CME(et, B, ur, er)


umin = ur(1); umax = ur(2);
% Cálculo do erro
%et = yref - y;
e = et / er;
if e < -1, e = -1;  elseif e > 1, e = 1; end
% Cálculo de u
if abs(e) == 1, ut = e; else ss = e - sign(e); ut = sign(ss) * (abs(ss) ^ (2 ^ -B) - 1); end
% Cálculo da saída
a = (umax - umin) / 2; u = a * (ut - 1) + umax;

end

== matlab function LQR - Keep Straight/CME2 ==
  data: u output double size=1; et input double size=1; B input double size=1; ur input double size=[2,1]; er input double size=1
% et: erro (ref-meas)
% B: Parâmetro 3
% ur: Parâmetro 2 (batentes do controle)
% er: Parâmetro
function u = CME(et, B, ur, er)


umin = ur(1); umax = ur(2);
% Cálculo do erro
%et = yref - y;
e = et / er;
if e < -1, e = -1;  elseif e > 1, e = 1; end
% Cálculo de u
if abs(e) == 1, ut = e; else ss = e - sign(e); ut = sign(ss) * (abs(ss) ^ (2 ^ -B) - 1); end
% Cálculo da saída
a = (umax - umin) / 2; u = a * (ut - 1) + umax;

end
